simulink model "aruco_guidance"  (R2017b)
settings: Solver=VariableStepAuto  StartTime=0.0  StopTime=10.0  RelTol=1e-3
undefined symbols (not defined in the file): Data, Data_SL_Info
libraries: dspstat3 x13, simulink x8, robotlib x2
settings Model: Creator=a  LastModifiedBy=a

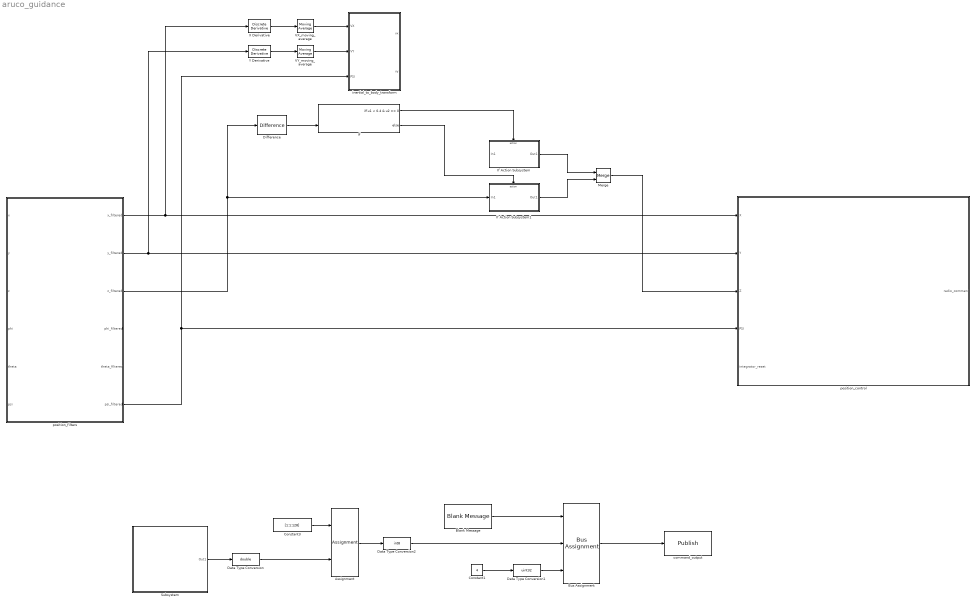
== system aruco_guidance ==
  " VX_moving_average" : dspstat3/Moving Average  Method=Sliding window  SpecifyWindowLength=on  WindowLength=5  ForgettingFactor=0.9  SimulateUsing=Code generation
  " VY_moving_average" : dspstat3/Moving Average  Method=Sliding window  SpecifyWindowLength=on  WindowLength=5  ForgettingFactor=0.9  SimulateUsing=Code generation
  Assignment : Assignment  DiagnosticForDimensions=Warning  IndexOptions=Index vector (dialog)  Indices=[1 2 3 4]  OutputSizes=1
  Blank Message : robotlib/Blank Message  SourceLibraryInfo=This block requires Robotics System Toolbox  messageType=std_msgs/Int8MultiArray  SampleTime=0.05
      settings: SourceProductBaseCode=RO
  Bus Assignment : BusAssignment  AssignedSignals=Data,Data_SL_Info.CurrentLength
  Constant1 : Constant  Value=4
  Constant3 : Constant  Value=[1:1:128]
  Data Type Conversion : DataTypeConversion  OutDataTypeStr=double
  Data Type Conversion1 : DataTypeConversion  OutDataTypeStr=uint32
  Data Type Conversion2 : DataTypeConversion  OutDataTypeStr=int8
  Difference : simulink/Discrete/Difference  ICPrevInput=0.0  OutMin=[]  OutMax=[]  OutDataType=fixdt(1, 16)  OutScaling=2^-10  DoSatur=off
  If : If  NumInputs=2  IfExpression=u1 < 0.4 & u2 == 0
  If Action Subsystem : Subsystem  TreatAsAtomicUnit=on
  If Action Subsystem1 : Subsystem  TreatAsAtomicUnit=on
  Merge : Merge
  Subsystem : Subsystem  mask{red=0.0, green=0.0, blue=15.0, enable=1}
  X Derivative : simulink/Discrete/Discrete Derivative  gainval=1.0  ICPrevScaledInput=0.0  OutMin=[]  OutMax=[]  OutDataType=fixdt(1, 16)  OutScaling=2^-10  DoSatur=off
  Y Derivative : simulink/Discrete/Discrete Derivative  gainval=1.0  ICPrevScaledInput=0.0  OutMin=[]  OutMax=[]  OutDataType=fixdt(1, 16)  OutScaling=2^-10  DoSatur=off
  "command_output " : robotlib/Publish  SourceLibraryInfo=This block requires Robotics System Toolbox  topicSource=Select from ROS network  topic=/quadrotor_1/LED  messageType=std_msgs/Int8MultiArray  messageQueueLength=1
      settings: SourceProductBaseCode=RO
  inertial_to_body_transform : Subsystem
  position_control : Subsystem
  position_filters : Subsystem
  wires:
  position_filters/6(psi_filtered) -> inertial_to_body_transform/3(PSI), position_control/4(PSI)
  If/2 -> If Action Subsystem1/Action
  X Derivative/1 -> " VX_moving_average"/1
  Merge/1 -> position_control/3(Z)
  position_filters/2(y_filtered) -> Y Derivative/1, position_control/2(Y)
  position_filters/1(x_filtered) -> X Derivative/1, position_control/1(X)
  position_filters/3(z_filtered) -> Difference/1, If Action Subsystem1/1(In1)
  " VY_moving_average"/1 -> inertial_to_body_transform/2(VY)
  If Action Subsystem1/1(Out1) -> Merge/2
  If/1 -> If Action Subsystem/Action
  Y Derivative/1 -> " VY_moving_average"/1
  If Action Subsystem/1(Out1) -> Merge/1
  " VX_moving_average"/1 -> inertial_to_body_transform/1(VX)
  ? -> If Action Subsystem/1(In1)
  Difference/1 -> If/2
  Blank Message/1 -> Bus Assignment/1
  Data Type Conversion2/1 -> Bus Assignment/2
  Bus Assignment/1 -> "command_output "/1
  Subsystem/1(Out1) -> Data Type Conversion/1
  Assignment/1 -> Data Type Conversion2/1
  Constant1/1 -> Data Type Conversion1/1
  Data Type Conversion1/1 -> Bus Assignment/3
  Data Type Conversion/1 -> Assignment/2
  Constant3/1 -> Assignment/1

== system aruco_guidance/If Action Subsystem ==
  In1 : Inport
  Action Port : ActionPort  ActionType=then
  Out1 : Outport
  wires:
  In1/1 -> Out1/1

== system aruco_guidance/If Action Subsystem1 ==
  In1 : Inport
  Action Port : ActionPort  ActionType=else
  Out1 : Outport
  wires:
  In1/1 -> Out1/1

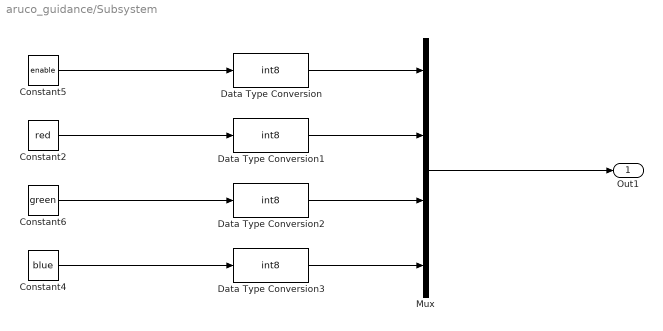
== system aruco_guidance/Subsystem ==
  Constant2 : Constant  Value=red
  Constant4 : Constant  Value=blue
  Constant5 : Constant  Value=enable
  Constant6 : Constant  Value=green
  Data Type Conversion{,1..3} (4 alike) : DataTypeConversion  OutDataTypeStr=int8
  Mux : Mux
  Out1 : Outport
  wires:
  Constant2/1 -> Data Type Conversion1/1
  Mux/1 -> Out1/1
  Constant5/1 -> Data Type Conversion/1
  Constant4/1 -> Data Type Conversion3/1
  Constant6/1 -> Data Type Conversion2/1
  Data Type Conversion/1 -> Mux/1
  Data Type Conversion1/1 -> Mux/2
  Data Type Conversion2/1 -> Mux/3
  Data Type Conversion3/1 -> Mux/4

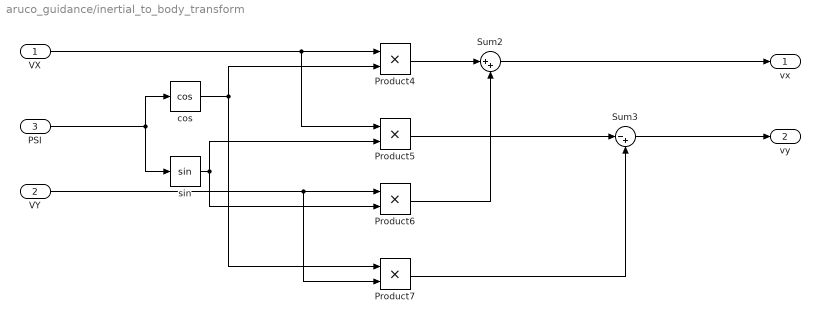
== system aruco_guidance/inertial_to_body_transform ==
  VX : Inport
  VY : Inport  Port=2
  PSI : Inport  Port=3
  Product{4..7} (4 alike) : Product
  Sum2 : Sum  Inputs=|++
  Sum3 : Sum  Inputs=|-+
  cos : Trigonometry  Operator=cos
  sin : Trigonometry
  vx : Outport
  vy : Outport  Port=2
  wires:
  Product5/1 -> Sum3/1
  PSI/1 -> sin/1, cos/1
  cos/1 -> Product7/1, Product4/2
  VY/1 -> Product7/2, Product6/1
  Sum3/1 -> vy/1
  sin/1 -> Product6/2, Product5/2
  VX/1 -> Product5/1, Product4/1
  Product6/1 -> Sum2/2
  Product7/1 -> Sum3/2
  Sum2/1 -> vx/1
  Product4/1 -> Sum2/1

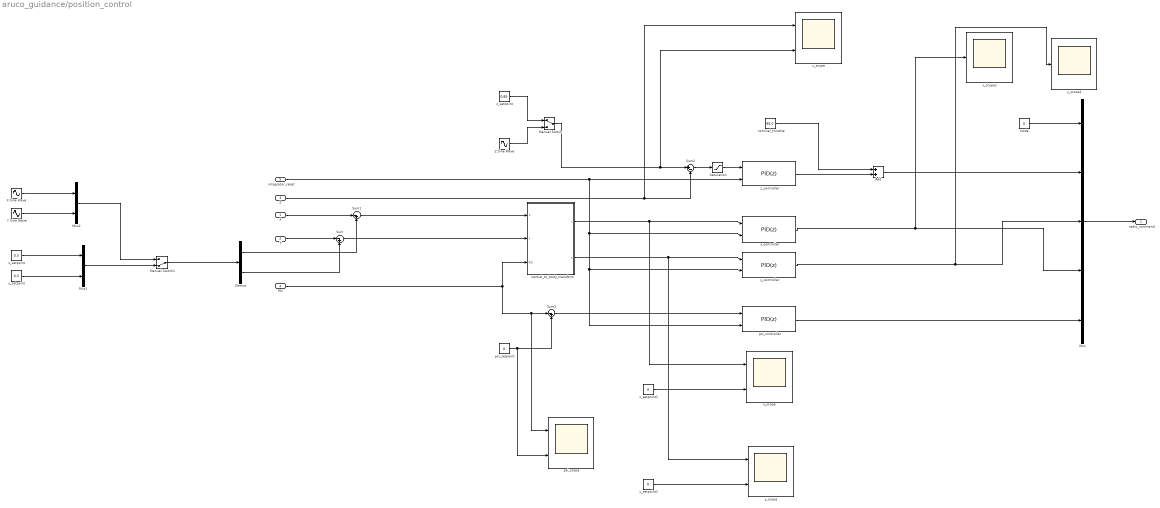
== system aruco_guidance/position_control ==
  X : Inport
  Y : Inport  Port=2
  Z : Inport  Port=3
  PSI : Inport  Port=4
  integrator_reset : Inport  Port=5
  Add : Sum
  Demux : Demux  Outputs=2
  Manual Switch : ManualSwitch
  Manual Switch1 : ManualSwitch  CurrentSetting=0
  Mux : Mux  Inputs=5
  Mux1 : Mux  Inputs=2
  Mux2 : Mux  Inputs=2
  Saturation : Saturate
  Sum : Sum  Inputs=|-+
  Sum1 : Sum  Inputs=|-+
  Sum2 : Sum  Inputs=|+-
  Sum3 : Sum  Inputs=|-+
  X Sine Wave : Sin  Amplitude=0.18  Bias=0.3  Frequency=0.8
  Y Sine Wave : Sin  Amplitude=0.18  Bias=0.3  Frequency=0.8  Phase=pi/2
  Z Sine Wave : Sin  Amplitude=0.1  Bias=0.85
  inertial_to_body_transform : Subsystem
  mode : Constant  Value=0
  nominal_throttle : Constant  Value=85.0
  psi_controller : simulink/Continuous/PID Controller  Controller=PID  TimeDomain=Discrete-time  SampleTime=-1  IntegratorMethod=Forward Euler  FilterMethod=Forward Euler  Form=Parallel  UseFilter=on  ControllerParametersSource=internal  P=-20  I=-2  D=-2  N=100  InitialConditionSource=internal  InitialConditionForIntegrator=0  InitialConditionForFilter=0  ExternalReset=either  LimitOutput=on  UpperSaturationLimit=120  LowerSaturationLimit=-120  LinearizeAsGain=off  AntiWindupMode=none  Kb=1  TrackingMode=off  Kt=1  PParamMin=[]  PParamMax=[]  IParamMin=[]  IParamMax=[]  DParamMin=[]  DParamMax=[]  NParamMin=[]  NParamMax=[]  KbParamMin=[]  KbParamMax=[]  KtParamMin=[]  KtParamMax=[]  POutMin=[]  POutMax=[]  IOutMin=[]  IOutMax=[]  DOutMin=[]  DOutMax=[]  NOutMin=[]  NOutMax=[]  KbOutMin=[]  KbOutMax=[]  KtOutMin=[]  KtOutMax=[]  IntegratorOutMin=[]  IntegratorOutMax=[]  FilterOutMin=[]  FilterOutMax=[]  SumOutMin=[]  SumOutMax=[]  SumI1OutMin=[]  SumI1OutMax=[]  SumI2OutMin=[]  SumI2OutMax=[]  SumI3OutMin=[]  SumI3OutMax=[]  SumDOutMin=[]  SumDOutMax=[]  SaturationOutMin=[]  SaturationOutMax=[]  IntegratorContinuousStateAttributes=''  IntegratorStateMustResolveToSignalObject=off  IntegratorRTWStateStorageClass=Auto  FilterContinuousStateAttributes=''  FilterStateMustResolveToSignalObject=off  FilterRTWStateStorageClass=Auto  DifferentiatorICPrevScaledInput=0  DifferentiatorOutMin=[]  DifferentiatorOutMax=[]  InitialConditionSetting=State (most efficient)  FilterDiffOutCoefMin=[]  FilterDiffOutCoefMax=[]  SumDenOutMin=[]  SumDenOutMax=[]  SumNumOutMin=[]  SumNumOutMax=[]  ReciprocalOutMin=[]  ReciprocalOutMax=[]  DivideOutMin=[]  DivideOutMax=[]  TunerSelectOption=Transfer Function Based (PID Tuner App)
  psi_scope : Scope  NumInputPorts=2
  psi_setpoint : Constant  Value=0
  x_controller : simulink/Continuous/PID Controller  Controller=PID  TimeDomain=Discrete-time  SampleTime=-1  IntegratorMethod=Forward Euler  FilterMethod=Forward Euler  Form=Parallel  UseFilter=on  ControllerParametersSource=internal  P=-47  I=-9  D=-20  N=100  InitialConditionSource=internal  InitialConditionForIntegrator=0  InitialConditionForFilter=0  ExternalReset=either  LimitOutput=on  UpperSaturationLimit=120  LowerSaturationLimit=-120  LinearizeAsGain=off  AntiWindupMode=none  Kb=1  TrackingMode=off  Kt=-10  PParamMin=[]  PParamMax=[]  IParamMin=[]  IParamMax=[]  DParamMin=[]  DParamMax=[]  NParamMin=[]  NParamMax=[]  KbParamMin=[]  KbParamMax=[]  KtParamMin=[]  KtParamMax=[]  POutMin=[]  POutMax=[]  IOutMin=[]  IOutMax=[]  DOutMin=[]  DOutMax=[]  NOutMin=[]  NOutMax=[]  KbOutMin=[]  KbOutMax=[]  KtOutMin=[]  KtOutMax=[]  IntegratorOutMin=[]  IntegratorOutMax=[]  FilterOutMin=[]  FilterOutMax=[]  SumOutMin=[]  SumOutMax=[]  SumI1OutMin=[]  SumI1OutMax=[]  SumI2OutMin=[]  SumI2OutMax=[]  SumI3OutMin=[]  SumI3OutMax=[]  SumDOutMin=[]  SumDOutMax=[]  SaturationOutMin=[]  SaturationOutMax=[]  IntegratorContinuousStateAttributes=''  IntegratorStateMustResolveToSignalObject=off  IntegratorRTWStateStorageClass=Auto  FilterContinuousStateAttributes=''  FilterStateMustResolveToSignalObject=off  FilterRTWStateStorageClass=Auto  DifferentiatorICPrevScaledInput=0  DifferentiatorOutMin=[]  DifferentiatorOutMax=[]  InitialConditionSetting=State (most efficient)  FilterDiffOutCoefMin=[]  FilterDiffOutCoefMax=[]  SumDenOutMin=[]  SumDenOutMax=[]  SumNumOutMin=[]  SumNumOutMax=[]  ReciprocalOutMin=[]  ReciprocalOutMax=[]  DivideOutMin=[]  DivideOutMax=[]  TunerSelectOption=Transfer Function Based (PID Tuner App)
  x_scope : Scope  NumInputPorts=2
  x_scope1 : Scope
  x_setpoint : Constant  Value=0.3
  x_setpoint1 : Constant  Value=0
  y_controller : simulink/Continuous/PID Controller  Controller=PID  TimeDomain=Discrete-time  SampleTime=-1  IntegratorMethod=Forward Euler  FilterMethod=Forward Euler  Form=Parallel  UseFilter=on  ControllerParametersSource=internal  P=-47  I=-9  D=-20  N=100  InitialConditionSource=internal  InitialConditionForIntegrator=0  InitialConditionForFilter=0  ExternalReset=either  LimitOutput=on  UpperSaturationLimit=120  LowerSaturationLimit=-120  LinearizeAsGain=off  AntiWindupMode=none  Kb=1  TrackingMode=off  Kt=-10  PParamMin=[]  PParamMax=[]  IParamMin=[]  IParamMax=[]  DParamMin=[]  DParamMax=[]  NParamMin=[]  NParamMax=[]  KbParamMin=[]  KbParamMax=[]  KtParamMin=[]  KtParamMax=[]  POutMin=[]  POutMax=[]  IOutMin=[]  IOutMax=[]  DOutMin=[]  DOutMax=[]  NOutMin=[]  NOutMax=[]  KbOutMin=[]  KbOutMax=[]  KtOutMin=[]  KtOutMax=[]  IntegratorOutMin=[]  IntegratorOutMax=[]  FilterOutMin=[]  FilterOutMax=[]  SumOutMin=[]  SumOutMax=[]  SumI1OutMin=[]  SumI1OutMax=[]  SumI2OutMin=[]  SumI2OutMax=[]  SumI3OutMin=[]  SumI3OutMax=[]  SumDOutMin=[]  SumDOutMax=[]  SaturationOutMin=[]  SaturationOutMax=[]  IntegratorContinuousStateAttributes=''  IntegratorStateMustResolveToSignalObject=off  IntegratorRTWStateStorageClass=Auto  FilterContinuousStateAttributes=''  FilterStateMustResolveToSignalObject=off  FilterRTWStateStorageClass=Auto  DifferentiatorICPrevScaledInput=0  DifferentiatorOutMin=[]  DifferentiatorOutMax=[]  InitialConditionSetting=State (most efficient)  FilterDiffOutCoefMin=[]  FilterDiffOutCoefMax=[]  SumDenOutMin=[]  SumDenOutMax=[]  SumNumOutMin=[]  SumNumOutMax=[]  ReciprocalOutMin=[]  ReciprocalOutMax=[]  DivideOutMin=[]  DivideOutMax=[]  TunerSelectOption=Transfer Function Based (PID Tuner App)
  y_scope : Scope  NumInputPorts=2
  y_scope1 : Scope
  y_setpoint : Constant  Value=0.3
  y_setpoint1 : Constant  Value=0
  z_controller : simulink/Continuous/PID Controller  Controller=PID  TimeDomain=Discrete-time  SampleTime=-1  IntegratorMethod=Forward Euler  FilterMethod=Forward Euler  Form=Parallel  UseFilter=on  ControllerParametersSource=internal  P=20  I=10  D=14  N=100  InitialConditionSource=internal  InitialConditionForIntegrator=0  InitialConditionForFilter=0  ExternalReset=either  LimitOutput=on  UpperSaturationLimit=35  LowerSaturationLimit=-85  LinearizeAsGain=off  AntiWindupMode=none  Kb=1  TrackingMode=off  Kt=1  PParamMin=[]  PParamMax=[]  IParamMin=[]  IParamMax=[]  DParamMin=[]  DParamMax=[]  NParamMin=[]  NParamMax=[]  KbParamMin=[]  KbParamMax=[]  KtParamMin=[]  KtParamMax=[]  POutMin=[]  POutMax=[]  IOutMin=[]  IOutMax=[]  DOutMin=[]  DOutMax=[]  NOutMin=[]  NOutMax=[]  KbOutMin=[]  KbOutMax=[]  KtOutMin=[]  KtOutMax=[]  IntegratorOutMin=[]  IntegratorOutMax=[]  FilterOutMin=[]  FilterOutMax=[]  SumOutMin=[]  SumOutMax=[]  SumI1OutMin=[]  SumI1OutMax=[]  SumI2OutMin=[]  SumI2OutMax=[]  SumI3OutMin=[]  SumI3OutMax=[]  SumDOutMin=[]  SumDOutMax=[]  SaturationOutMin=[]  SaturationOutMax=[]  IntegratorContinuousStateAttributes=''  IntegratorStateMustResolveToSignalObject=off  IntegratorRTWStateStorageClass=Auto  FilterContinuousStateAttributes=''  FilterStateMustResolveToSignalObject=off  FilterRTWStateStorageClass=Auto  DifferentiatorICPrevScaledInput=0  DifferentiatorOutMin=[]  DifferentiatorOutMax=[]  InitialConditionSetting=State (most efficient)  FilterDiffOutCoefMin=[]  FilterDiffOutCoefMax=[]  SumDenOutMin=[]  SumDenOutMax=[]  SumNumOutMin=[]  SumNumOutMax=[]  ReciprocalOutMin=[]  ReciprocalOutMax=[]  DivideOutMin=[]  DivideOutMax=[]  TunerSelectOption=Transfer Function Based (PID Tuner App)
  z_scope : Scope  NumInputPorts=2
  z_setpoint : Constant  Value=0.85
  radio_command : Outport
  wires:
  Z/1 -> z_scope/1, Sum2/2
  nominal_throttle/1 -> Add/1
  z_controller/1 -> Add/2
  Sum2/1 -> Saturation/1
  Manual Switch/1 -> z_scope/2, Sum2/1
  integrator_reset/1 -> psi_controller/2, y_controller/2, x_controller/2, z_controller/2
  Y/1 -> Sum/1
  X/1 -> Sum1/1
  psi_controller/1 -> Mux/5
  y_controller/1 -> Mux/3, y_scope1/1
  PSI/1 -> psi_scope/1, Sum3/1, inertial_to_body_transform/3(PSI)
  x_controller/1 -> x_scope1/1, Mux/4
  y_setpoint/1 -> Mux1/2
  Sum/1 -> inertial_to_body_transform/2(Y)
  Sum1/1 -> inertial_to_body_transform/1(X)
  x_setpoint/1 -> Mux1/1
  Add/1 -> Mux/2
  mode/1 -> Mux/1
  Mux/1 -> radio_command/1
  x_setpoint1/1 -> x_scope/2
  y_setpoint1/1 -> y_scope/2
  inertial_to_body_transform/1(x) -> x_scope/1, x_controller/1
  inertial_to_body_transform/2(y) -> y_scope/1, y_controller/1
  psi_setpoint/1 -> psi_scope/2, Sum3/2
  Sum3/1 -> psi_controller/1
  z_setpoint/1 -> Manual Switch/1
  Z Sine Wave/1 -> Manual Switch/2
  Mux1/1 -> Manual Switch1/2
  Demux/1 -> Sum1/2
  Demux/2 -> Sum/2
  Y Sine Wave/1 -> Mux2/2
  X Sine Wave/1 -> Mux2/1
  Mux2/1 -> Manual Switch1/1
  Manual Switch1/1 -> Demux/1
  Saturation/1 -> z_controller/1

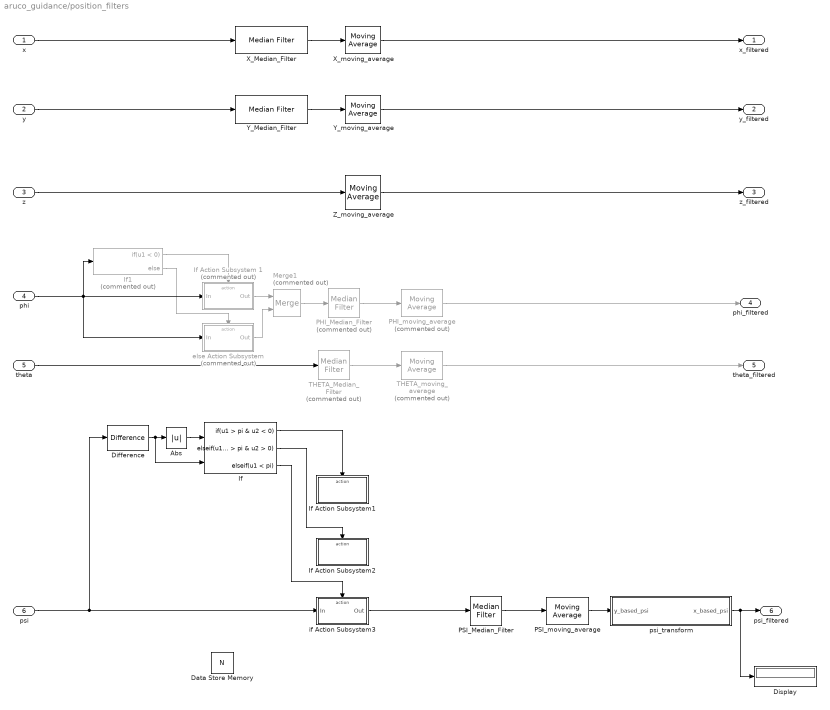
== system aruco_guidance/position_filters ==
  x : Inport
  y : Inport  Port=2
  z : Inport  Port=3
  phi : Inport  Port=4
  theta : Inport  Port=5
  psi : Inport  Port=6
  " PHI_moving_average" : dspstat3/Moving Average  Commented=on  Method=Sliding window  SpecifyWindowLength=on  WindowLength=30  ForgettingFactor=0.9  SimulateUsing=Code generation
  " PSI_moving_average" : dspstat3/Moving Average  Method=Sliding window  SpecifyWindowLength=on  WindowLength=30  ForgettingFactor=0.9  SimulateUsing=Code generation
  " THETA_moving_average" : dspstat3/Moving Average  Commented=on  Method=Sliding window  SpecifyWindowLength=on  WindowLength=30  ForgettingFactor=0.9  SimulateUsing=Code generation
  " X_moving_average" : dspstat3/Moving Average  Method=Sliding window  SpecifyWindowLength=on  WindowLength=30  ForgettingFactor=0.9  SimulateUsing=Code generation
  " Y_moving_average" : dspstat3/Moving Average  Method=Sliding window  SpecifyWindowLength=on  WindowLength=30  ForgettingFactor=0.9  SimulateUsing=Code generation
  Abs : Abs
  Data Store Memory : DataStoreMemory  DataStoreName=N  ReadBeforeWriteMsg=warning  WriteAfterWriteMsg=warning  WriteAfterReadMsg=warning  ShowAdditionalParam=off  OutDataTypeStr=int32
  Difference : simulink/Discrete/Difference  ICPrevInput=0.0  OutMin=[]  OutMax=[]  OutDataType=fixdt(1, 16)  OutScaling=2^-10  DoSatur=off
  Display : Display
  If : If  NumInputs=2  IfExpression=u1 > pi & u2 < 0  ElseIfExpressions=u1 > pi & u2 > 0 , u1 < pi  ShowElse=off
  If Action Subsystem 1 : Subsystem  Commented=on  TreatAsAtomicUnit=on
  If Action Subsystem1 : Subsystem  TreatAsAtomicUnit=on
  If Action Subsystem2 : Subsystem  TreatAsAtomicUnit=on
  If1 : If  Commented=on  IfExpression=u1 < 0
  Merge1 : Merge  Commented=on
  PHI_Median_Filter : dspstat3/Median Filter  Commented=on  WindowLength=10  SimulateUsing=Interpreted execution
      settings: SourceProductName=DSP System Toolbox  SourceProductBaseCode=DS
  PSI_Median_Filter : dspstat3/Median Filter  WindowLength=10  SimulateUsing=Interpreted execution
      settings: SourceProductName=DSP System Toolbox  SourceProductBaseCode=DS
  THETA_Median_Filter : dspstat3/Median Filter  Commented=on  WindowLength=10  SimulateUsing=Interpreted execution
      settings: SourceProductName=DSP System Toolbox  SourceProductBaseCode=DS
  X_Median_Filter : dspstat3/Median Filter  WindowLength=10  SimulateUsing=Interpreted execution
      settings: SourceProductName=DSP System Toolbox  SourceProductBaseCode=DS
  Y_Median_Filter : dspstat3/Median Filter  WindowLength=10  SimulateUsing=Interpreted execution
      settings: SourceProductName=DSP System Toolbox  SourceProductBaseCode=DS
  Z_moving_average : dspstat3/Moving Average  Method=Sliding window  SpecifyWindowLength=on  WindowLength=20  ForgettingFactor=0.9  SimulateUsing=Code generation
  else Action Subsystem : Subsystem  Commented=on  TreatAsAtomicUnit=on
  if Action Subsystem3 : Subsystem  TreatAsAtomicUnit=on
  psi_transform : Subsystem
  x_filtered : Outport
  y_filtered : Outport  Port=2
  z_filtered : Outport  Port=3
  phi_filtered : Outport  Port=4
  theta_filtered : Outport  Port=5
  psi_filtered : Outport  Port=6
  wires:
  x/1 -> X_Median_Filter/1
  y/1 -> Y_Median_Filter/1
  Y_Median_Filter/1 -> " Y_moving_average"/1
  THETA_Median_Filter/1 -> " THETA_moving_average"/1
  else Action Subsystem/1(Out) -> Merge1/2
  PSI_Median_Filter/1 -> " PSI_moving_average"/1
  " Y_moving_average"/1 -> y_filtered/1
  If Action Subsystem 1/1(Out) -> Merge1/1
  " X_moving_average"/1 -> x_filtered/1
  " THETA_moving_average"/1 -> theta_filtered/1
  X_Median_Filter/1 -> " X_moving_average"/1
  psi_transform/1(x_based_psi) -> Display/1, psi_filtered/1
  " PSI_moving_average"/1 -> psi_transform/1(y_based_psi)
  If1/2 -> else Action Subsystem/Action
  phi/1 -> If1/1, else Action Subsystem/1(In), If Action Subsystem 1/1(In)
  theta/1 -> THETA_Median_Filter/1
  " PHI_moving_average"/1 -> phi_filtered/1
  PHI_Median_Filter/1 -> " PHI_moving_average"/1
  If1/1 -> If Action Subsystem 1/Action
  Merge1/1 -> PHI_Median_Filter/1
  z/1 -> Z_moving_average/1
  Z_moving_average/1 -> z_filtered/1
  If/3 -> if Action Subsystem3/Action
  If/1 -> If Action Subsystem1/Action
  psi/1 -> Difference/1, if Action Subsystem3/1(In)
  if Action Subsystem3/1(Out) -> PSI_Median_Filter/1
  Difference/1 -> If/2, Abs/1
  Abs/1 -> If/1
  If/2 -> If Action Subsystem2/Action

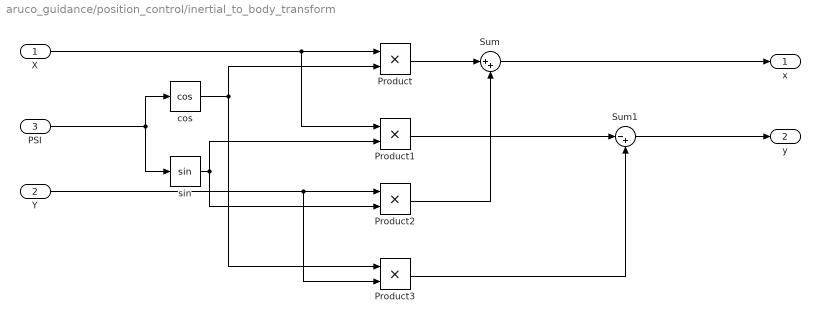
== system aruco_guidance/position_control/inertial_to_body_transform ==
  X : Inport
  Y : Inport  Port=2
  PSI : Inport  Port=3
  Product{,1..3} (4 alike) : Product
  Sum : Sum  Inputs=|++
  Sum1 : Sum  Inputs=|-+
  cos : Trigonometry  Operator=cos
  sin : Trigonometry
  x : Outport
  y : Outport  Port=2
  wires:
  sin/1 -> Product2/2, Product1/2
  Product3/1 -> Sum1/2
  Sum/1 -> x/1
  Product/1 -> Sum/1
  Y/1 -> Product3/2, Product2/1
  PSI/1 -> sin/1, cos/1
  X/1 -> Product1/1, Product/1
  Sum1/1 -> y/1
  cos/1 -> Product3/1, Product/2
  Product2/1 -> Sum/2
  Product1/1 -> Sum1/1

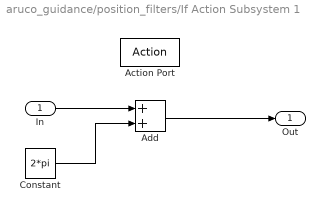
== system aruco_guidance/position_filters/If Action Subsystem 1 ==
  In : Inport
  Action Port : ActionPort
  Add : Sum
  Constant : Constant  Value=2*pi
  Out : Outport
  wires:
  Constant/1 -> Add/2
  Add/1 -> Out/1
  In/1 -> Add/1

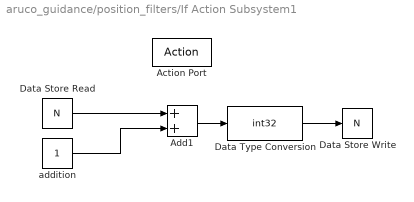
== system aruco_guidance/position_filters/If Action Subsystem1 ==
  Action Port : ActionPort
  Add1 : Sum
  Data Store Read : DataStoreRead  DataStoreName=N
  Data Store Write : DataStoreWrite  DataStoreName=N
  Data Type Conversion : DataTypeConversion  OutDataTypeStr=int32
  addition : Constant
  wires:
  Data Store Read/1 -> Add1/1
  addition/1 -> Add1/2
  Add1/1 -> Data Type Conversion/1
  Data Type Conversion/1 -> Data Store Write/1

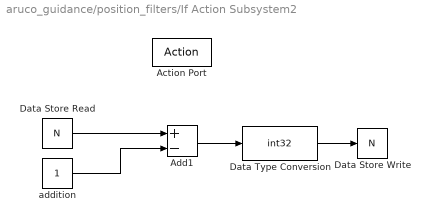
== system aruco_guidance/position_filters/If Action Subsystem2 ==
  Action Port : ActionPort
  Add1 : Sum  Inputs=+-
  Data Store Read : DataStoreRead  DataStoreName=N
  Data Store Write : DataStoreWrite  DataStoreName=N
  Data Type Conversion : DataTypeConversion  OutDataTypeStr=int32
  addition : Constant
  wires:
  addition/1 -> Add1/2
  Data Store Read/1 -> Add1/1
  Add1/1 -> Data Type Conversion/1
  Data Type Conversion/1 -> Data Store Write/1

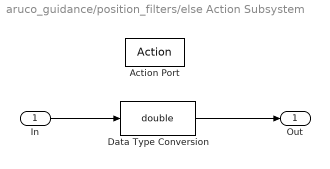
== system aruco_guidance/position_filters/else Action Subsystem ==
  In : Inport
  Action Port : ActionPort
  Data Type Conversion : DataTypeConversion  OutDataTypeStr=double
  Out : Outport
  wires:
  Data Type Conversion/1 -> Out/1
  In/1 -> Data Type Conversion/1

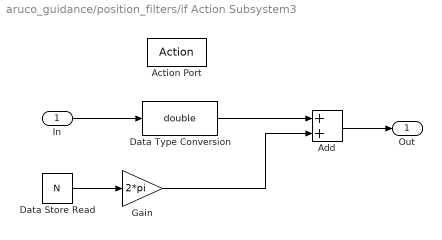
== system aruco_guidance/position_filters/if Action Subsystem3 ==
  In : Inport
  Action Port : ActionPort
  Add : Sum
  Data Store Read : DataStoreRead  DataStoreName=N
  Data Type Conversion : DataTypeConversion  OutDataTypeStr=double
  Gain : Gain  Gain=2*pi
  Out : Outport
  wires:
  Data Type Conversion/1 -> Add/1
  In/1 -> Data Type Conversion/1
  Data Store Read/1 -> Gain/1
  Gain/1 -> Add/2
  Add/1 -> Out/1

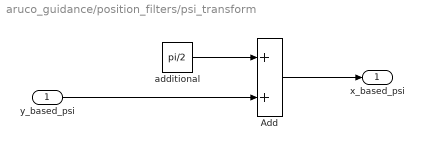
== system aruco_guidance/position_filters/psi_transform ==
  y_based_psi : Inport
  Add : Sum
  additional : Constant  Value=pi/2
  x_based_psi : Outport
  wires:
  y_based_psi/1 -> Add/2
  Add/1 -> x_based_psi/1
  additional/1 -> Add/1
